simulink model "Simulink_model"  (R2017b)
settings: Solver=VariableStepAuto  StartTime=0.0  StopTime=10.0  RelTol=1e-3
settings Model: Creator=LUCIA  LastModifiedBy=LUCIA

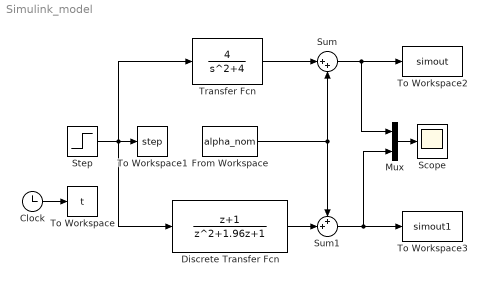
== system Simulink_model ==
  Clock : Clock
  Discrete Transfer Fcn : DiscreteTransferFcn  Numerator=[1 1]  Denominator=[1 1.96 1]
  From Workspace : FromWorkspace  VariableName=alpha_nom  SampleTime=0
  Mux : Mux  Inputs=2
  Scope : Scope
  Step : Step  After=8  SampleTime=0
  Sum : Sum  Inputs=|++
  Sum1 : Sum  Inputs=++|
  To Workspace : ToWorkspace  VariableName=t  SaveFormat=Timeseries  SampleTime=-1
  To Workspace1 : ToWorkspace  VariableName=step  SaveFormat=Timeseries  SampleTime=-1
  To Workspace2 : ToWorkspace  VariableName=simout  SaveFormat=Timeseries  SampleTime=-1
  To Workspace3 : ToWorkspace  VariableName=simout1  SaveFormat=Timeseries  SampleTime=-1
  Transfer Fcn : TransferFcn  Numerator=4  Denominator=[1 0 4]
  wires:
  Clock/1 -> To Workspace/1
  Transfer Fcn/1 -> Sum/1
  From Workspace/1 -> Sum1/1, Sum/2
  Discrete Transfer Fcn/1 -> Sum1/2
  Step/1 -> Discrete Transfer Fcn/1, Transfer Fcn/1, To Workspace1/1
  Sum/1 -> Mux/1, To Workspace2/1
  Sum1/1 -> Mux/2, To Workspace3/1
  Mux/1 -> Scope/1
